simulink model "power_turbine_period2_1110_plots"  (R2025b)
settings: Solver=VariableStepAuto  StartTime=0.0  StopTime=100  RelTol=1e-3
undefined symbols (not defined in the file or in its folder): D1, Delta
libraries: spsThreePhaseBreakerLib x5, spsThreePhaseParallelRLCLoadLib x4, spsThreePhaseDynamicLoadLib x3, spsThreePhasePISectionLineLib x2, spsExcitationSystemLib x1, spsHydraulicTurbineandGovernorLib x1, spsLoadFlowBusLib x1, spsSynchronousMachinepuStandardLib x1, spsThreePhaseVIMeasurementLib x1, spsThreePhaseFaultLib x1, spsThreePhaseTransformerTwoWindingsLib x1, spsVoltageMeasurementLib x1
settings Model: Creator=Amaya  LastModifiedBy=Amaya

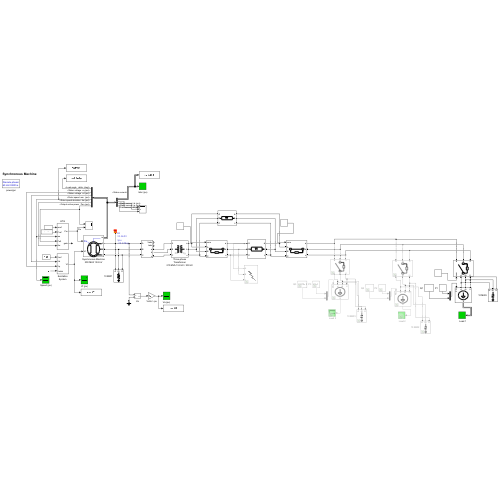
[thumbnail: Simulink's stored preview of the top-level diagram]
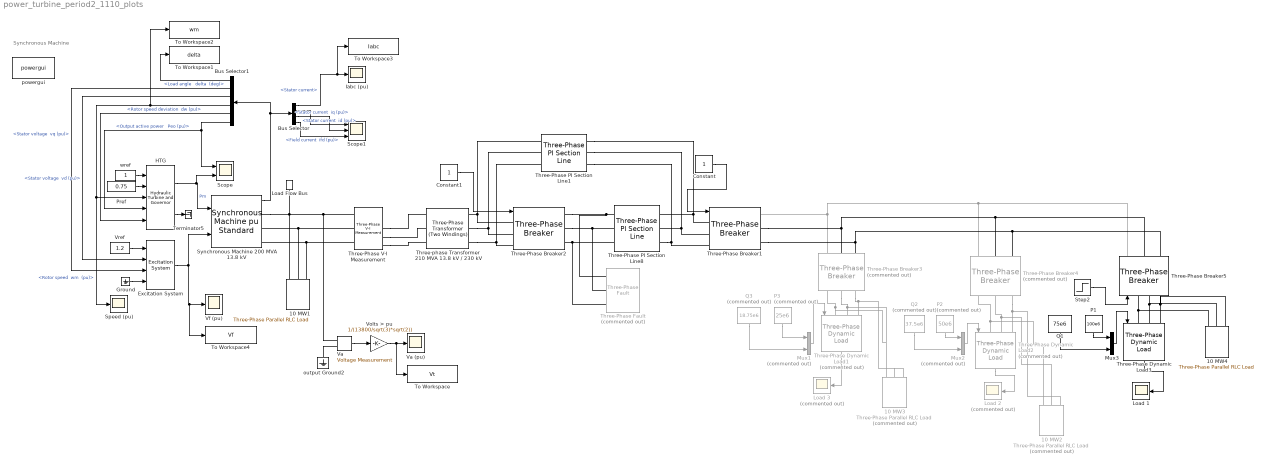
== system power_turbine_period2_1110_plots ==
  note: Synchronous Machine
  "  Load 1" : Scope
      settings: TimeSpan=2  ActiveDisplayYMinimum=-1.249999884558E+7  ActiveDisplayYMaximum=1.1249999987173E+8  DataLoggingVariableName=ScopeData3  DataLoggingSaveFormat=Array
  "  Load 2" : Scope  Commented=on
      settings: TimeSpan=2  ActiveDisplayYMinimum=-1.25E+7  ActiveDisplayYMaximum=1.125E+8  DataLoggingSaveFormat=Array
  "  Load 3" : Scope  Commented=on
      settings: TimeSpan=2  ActiveDisplayYMinimum=-1.25E+7  ActiveDisplayYMaximum=1.125E+8  DataLoggingVariableName=ScopeData2  DataLoggingSaveFormat=Array
  " Iabc (pu)" : Scope
      settings: TimeSpan=2  ActiveDisplayYMinimum=0.37186  ActiveDisplayYMaximum=0.41748  DataLoggingSaveFormat=Array
  " Speed (pu)" : Scope
      settings: TimeSpan=2  ActiveDisplayYMinimum=0.96201  ActiveDisplayYMaximum=1.29502  DataLoggingVariableName=ScopeData2  DataLoggingSaveFormat=Array
  10 MW1 : spsThreePhaseParallelRLCLoadLib/Three-Phase Parallel RLC Load  LConnTagsString=A|B|C  Configuration=Y (grounded)  NominalVoltage=230e3  Vabc=[1e3 1e3 1e3]  Vabcp=[1e3 1e3 1e3]  NominalFrequency=60  UnbalancedPower=off  ActivePower=5e6  InductivePower=0  CapacitivePower=0  Pabc=[10e3 9e3 11e3]  QLabc=[100 90 110]  QCabc=[100 90 110]  Pabcp=[10e3 9e3 11e3]  QLabcp=[100 90 110]  QCabcp=[100 90 110]  Measurements=None  LoadType=constant Z
  10 MW2 : spsThreePhaseParallelRLCLoadLib/Three-Phase Parallel RLC Load  Commented=on  LConnTagsString=A|B|C  Configuration=Y (grounded)  NominalVoltage=230e3  Vabc=[1e3 1e3 1e3]  Vabcp=[1e3 1e3 1e3]  NominalFrequency=60  UnbalancedPower=off  ActivePower=0  InductivePower=0  CapacitivePower=18.44e6  Pabc=[10e3 9e3 11e3]  QLabc=[100 90 110]  QCabc=[100 90 110]  Pabcp=[10e3 9e3 11e3]  QLabcp=[100 90 110]  QCabcp=[100 90 110]  Measurements=None  LoadType=constant Z
  10 MW3 : spsThreePhaseParallelRLCLoadLib/Three-Phase Parallel RLC Load  Commented=on  LConnTagsString=A|B|C  Configuration=Y (grounded)  NominalVoltage=230e3  Vabc=[1e3 1e3 1e3]  Vabcp=[1e3 1e3 1e3]  NominalFrequency=60  UnbalancedPower=off  ActivePower=0  InductivePower=0  CapacitivePower=9.21e6  Pabc=[10e3 9e3 11e3]  QLabc=[100 90 110]  QCabc=[100 90 110]  Pabcp=[10e3 9e3 11e3]  QLabcp=[100 90 110]  QCabcp=[100 90 110]  Measurements=None  LoadType=constant Z
  10 MW4 : spsThreePhaseParallelRLCLoadLib/Three-Phase Parallel RLC Load  LConnTagsString=A|B|C  Configuration=Y (grounded)  NominalVoltage=230e3  Vabc=[1e3 1e3 1e3]  Vabcp=[1e3 1e3 1e3]  NominalFrequency=60  UnbalancedPower=off  ActivePower=0  InductivePower=0  CapacitivePower=36.87e6  Pabc=[10e3 9e3 11e3]  QLabc=[100 90 110]  QCabc=[100 90 110]  Pabcp=[10e3 9e3 11e3]  QLabcp=[100 90 110]  QCabcp=[100 90 110]  Measurements=None  LoadType=constant Z
  Bus Selector : BusSelector  OutputSignals="Stator current,dq0 components.Stator current  id (pu),dq0 components.Stator current  iq (pu),dq0 components.Field current  ifd (pu)"
  Bus Selector1 : BusSelector  OutputSignals="Load angle   delta  (deg),dq0 components.Stator voltage  vq (pu),dq0 components.Stator voltage  vd (pu),Mechanical.Rotor speed  wm  (pu),Mechanical.Rotor speed deviation  dw (pu),Output active power   Peo (pu)"
  Constant : Constant
  Constant1 : Constant
  Excitation System : spsExcitationSystemLib/Excitation System  tr=20e-3  reg=[ 300, 0.001 ]  exc=[ 1, 0 ]  tgr=[ 0, 0 ]  damp=[ 0.001, 0.1 ]  sat=[ 0, 0 ]  lim=[ -1000, 1000, 0 ]  v0=[1,1.29071]
  Ground : Ground
  HTG : spsHydraulicTurbineandGovernorLib/Hydraulic Turbine and Governor  sm="[ 10/3  0.07 ]"  gate="[  0.01  0.97518  -0.1  0.1 ]"  reg="[  0.05  1.163  0.105  0  0.01  ]"  hyd="[  0  2.67  ]"  dref=0  po=0.751606
  Load Flow Bus : spsLoadFlowBusLib/Load Flow Bus  LConnTagsString=a  Phases=single  Connectors=on one side  ID=B1  Vbase=13.8e3  Vref=1  Vangle=0  VLF=1  VLFb=1  VLFc=1  angleLF=-23.67  angleLFb=0  angleLFc=0
      settings: AttributesFormatString=%<ID>\n%<Vbase>V\n%<VLF>pu\n%<angleLF>deg.
  Mux1 : Mux  Commented=on  Inputs=2
  Mux2 : Mux  Commented=on  Inputs=2
  Mux3 : Mux  Inputs=2
  P1 : Constant  Value=100e6
  P2 : Constant  Commented=on  Value=50e6
  P3 : Constant  Commented=on  Value=25e6
  Pref : Constant  Value=0.75
  Q1 : Constant  Value=75e6
  Q2 : Constant  Commented=on  Value=37.5e6
  Q3 : Constant  Commented=on  Value=18.75e6
  Scope : Scope  NumInputPorts=2
      settings: ActiveDisplayYMinimum=-11.7999  ActiveDisplayYMaximum=2.34274  DataLoggingVariableName=ScopeData4
  Scope1 : Scope  NumInputPorts=3
      settings: ActiveDisplayYMinimum=-1.06949  ActiveDisplayYMaximum=2.5715  DataLoggingVariableName=ScopeData4
  Step2 : Step  Time=0  SampleTime=0
  Synchronous Machine 200 MVA 13.8 kV : spsSynchronousMachinepuStandardLib/Synchronous Machine pu Standard  PresetModel=No  MechanicalLoad=Mechanical power Pm  ShowDetailedParameters=on  RotorType=Salient-pole  Units=per unit standard parameters  MeasurementBus=off  NominalParameters="[ 250E6  13800   60 ]"  Reactances1=[ 31 32 33 34 35 36 37 ]  Reactances2=[ 1.305, 0.296, 0.252, 0.474, 0.243, 0.18 ]  dAxisTimeConstants=Short-circuit  qAxisTimeConstants=Open-circuit  TimeConstants1=[]  TimeConstants2=[]  TimeConstants3=[]  TimeConstants4=[]  TimeConstants5=[ 1.01, 0.053, 0.1 ]  TimeConstants6=[]  TimeConstants7=[]  TimeConstants8=[]  StatorResistance=2.8544e-3  Mechanical=[ 3.2 0 2]  PolePairs=2  InitialConditions=[0 -94.2826 0.750185 0.750185 0.750185 -24.943 -144.943 95.057 1.29071]  SetSaturation=off  Saturation=[0.6404,0.7127,0.8441,0.9214,0.9956,1.082,1.19,1.316,1.457;0.7,0.7698,0.8872,0.9466,0.9969,1.046,1.1,1.151,1.201]  LoadFlowParameters=[1 150000000 0 0]  TsPowergui=0  TsBlock=-1  IterativeModel=Trapezoidal non iterative  IterativeDiscreteModel=Trapezoidal non iterative  BusType=PV  Pref=150000000  Qref=0  Qmin=-Inf  Qmax=Inf  PLF=0  QLF=0
  Terminator5 : Terminator
  Three-Phase Dynamic Load1 : spsThreePhaseDynamicLoadLib/Three-Phase Dynamic Load  Commented=on  NominalVoltage=[ 230e3 60 ]  ActiveReactivePowers=[25e6 18.75e6]  PositiveSequence=[0.994 -11.8]  ExternalControl=on  NpNq=[1.3 2]  TimeConstants="[0  0  0  0]"  MinimumVoltage=0.7  Tfilter=1e-4  LoadFlowParameters=[4,0,0,0,0]
      settings: LibrarySourceBlock=|
      | sps_lib/Passives/Three-Phase
      | Dynamic Load
  Three-Phase Dynamic Load2 : spsThreePhaseDynamicLoadLib/Three-Phase Dynamic Load  Commented=on  NominalVoltage=[ 230e3 60 ]  ActiveReactivePowers=[50e6 37.5e6]  PositiveSequence=[0.994 -11.8]  ExternalControl=on  NpNq=[1.3 2]  TimeConstants="[0  0  0  0]"  MinimumVoltage=0.7  Tfilter=1e-4  LoadFlowParameters=[4,0,0,0,0]
      settings: LibrarySourceBlock=|
      | sps_lib/Passives/Three-Phase
      | Dynamic Load
  Three-Phase Dynamic Load3 : spsThreePhaseDynamicLoadLib/Three-Phase Dynamic Load  NominalVoltage=[ 230e3 60 ]  ActiveReactivePowers=[100e6 75e6]  PositiveSequence=[0.994 -11.8]  ExternalControl=on  NpNq=[1.3 2]  TimeConstants="[0  0  0  0]"  MinimumVoltage=0.7  Tfilter=1e-4  LoadFlowParameters=[4,0,0,0,0]
      settings: LibrarySourceBlock=|
      | sps_lib/Passives/Three-Phase
      | Dynamic Load
  Three-Phase PI Section Line1 : spsThreePhasePISectionLineLib/Three-Phase PI Section Line  LConnTagsString=a|b|c  RConnTagsString=A|B|C  Length=125  Frequency=50  Resistances=[ 0.01273 0.3864]  Inductances="[ 0.9337e-3  4.1264e-3]"  Capacitances=[12.74e-9 7.751e-9]
  Three-Phase PI Section Line8 : spsThreePhasePISectionLineLib/Three-Phase PI Section Line  LConnTagsString=a|b|c  RConnTagsString=A|B|C  Length=125  Frequency=60  Resistances=[ 0.01273 0.3864]  Inductances="[ 0.9337e-3  4.1264e-3]"  Capacitances=[12.74e-9 7.751e-9]
  Three-Phase V-I Measurement : spsThreePhaseVIMeasurementLib/Three-Phase V-I Measurement  VoltageMeasurement=phase-to-ground  SetLabelV=off  LabelV=Vabc  Vpu=off  VpuLL=off  CurrentMeasurement=yes  SetLabelI=off  LabelI=Iabc  Ipu=off  Pbase=100e6  Vbase=500e3  OutputType=Complex  PhasorSimulation=on  PSBequivalent=0
  Three-Phase Breaker1 : spsThreePhaseBreakerLib/Three-Phase Breaker  InitialState=closed  SwitchA=on  SwitchB=on  SwitchC=on  SwitchTimes=[70.1 70+121/60]  External=on  BreakerResistance=0.01  SnubberResistance=1e6  SnubberCapacitance=inf  Measurements=None
  Three-Phase Breaker2 : spsThreePhaseBreakerLib/Three-Phase Breaker  InitialState=closed  SwitchA=on  SwitchB=on  SwitchC=on  SwitchTimes=[70.05 70.05+121/60]  External=on  BreakerResistance=0.01  SnubberResistance=1e6  SnubberCapacitance=inf  Measurements=None
  Three-Phase Breaker3 : spsThreePhaseBreakerLib/Three-Phase Breaker  Commented=on  InitialState=open  SwitchA=on  SwitchB=on  SwitchC=on  SwitchTimes=[100]  External=off  BreakerResistance=0.01  SnubberResistance=1e6  SnubberCapacitance=inf  Measurements=None
  Three-Phase Breaker4 : spsThreePhaseBreakerLib/Three-Phase Breaker  Commented=on  InitialState=open  SwitchA=on  SwitchB=on  SwitchC=on  SwitchTimes=[50]  External=off  BreakerResistance=0.01  SnubberResistance=1e6  SnubberCapacitance=inf  Measurements=None
  Three-Phase Breaker5 : spsThreePhaseBreakerLib/Three-Phase Breaker  InitialState=open  SwitchA=on  SwitchB=on  SwitchC=on  SwitchTimes="[7/60  121/60]"  External=on  BreakerResistance=0.01  SnubberResistance=1e6  SnubberCapacitance=inf  Measurements=None
  Three-Phase Fault : spsThreePhaseFaultLib/Three-Phase Fault  Commented=on  InitialStates=0  FaultA=on  FaultB=on  FaultC=on  GroundFault=on  SwitchTimes=[70 70.1]  External=off  SwitchStatus=NaN  FaultResistance=0.001  GroundResistance=1  SnubberResistance=1e6  SnubberCapacitance=inf  Measurements=None
  Three-phase Transformer 210 MVA 13.8 kV / 230 kV : spsThreePhaseTransformerTwoWindingsLib/Three-Phase Transformer (Two Windings)  Winding1Connection=Delta (D1)  Winding2Connection=Yg  CoreType=Three single-phase transformers  SetSaturation=off  Hysteresis=off  DataFile='hysteresis'  SetInitialFlux=off  Measurements=None  UNITS=pu  NominalPower=[ 210e6 60 ]  Winding1="[ 13.8e3 0.0027  0.08]"  Winding2=[ 230e3 0.0027 0.08]  Rm=500  Lm=500  L0=0.5  Saturation="[ 0,0  ;  0.005,1.2  ;  1.0,1.4 ]"  InitialFluxes=[ 0.8 , -0.8 , 0.7 ]  BreakLoop=off  DiscreteSolver=Trapezoidal iterative  DataType=off  TransfoNumber=0
  To Workspace : ToWorkspace  VariableName=Vt  SaveFormat=Structure With Time  SampleTime=-1
  To Workspace1 : ToWorkspace  VariableName=delta  SaveFormat=Structure With Time  SampleTime=-1
  To Workspace2 : ToWorkspace  VariableName=wm  SaveFormat=Structure With Time  SampleTime=-1
  To Workspace3 : ToWorkspace  VariableName=Iabc  SaveFormat=Structure With Time  SampleTime=-1
  To Workspace4 : ToWorkspace  VariableName=Vf  SaveFormat=Structure With Time  SampleTime=-1
  Va : spsVoltageMeasurementLib/Voltage Measurement  Tag=PoWeRsYsTeMmEaSuReMeNt  PhasorSimulation=on  OutputType=Magnitude  PSBequivalent=0
  Va (pu) : Scope
      settings: TimeSpan=2  ActiveDisplayYMinimum=0.99758  ActiveDisplayYMaximum=1.29648  DataLoggingVariableName=ScopeData3  DataLoggingSaveFormat=Array
  Vf (pu) : Scope
      settings: TimeSpan=2  ActiveDisplayYMinimum=-5.63103  ActiveDisplayYMaximum=28.67601  DataLoggingSaveFormat=Array
  Volts > pu : Gain  Gain=1/(13800/sqrt(3)*sqrt(2))  SaturateOnIntegerOverflow=on  OutDataTypeStr=Inherit: Same as input  ParamDataTypeStr=Inherit: Same as input
  Vref : Constant  Value=1.2
  output Ground2 : spsGroundLib/Ground  LConnTagsString=a
  powergui : spspowerguiLib/powergui  Priority=2  SimulationMode=Discrete phasor  SampleTime=50e-5  frequency=60  Iterations=50  frequencyindice=60  Pbase=100e6  ErrMax=0.0001  UnitsV=kV  UnitsW=MW  buscounter=0  FunctionMessages=off  echomessages=off  EnableUseOfTLC=off  CurrentSourceSwitches=off  DisableSnubberDevices=off  DisableRonSwitches=off  DisableVfSwitches=off  DisplayEquations=off  AutomaticDiscreteSolvers=off  SolverType=Tustin  Interpol=off  ExternalGateDelay=off  methode=off  Ts=0  x0status=blocks  SPID=on  SwTol=0  HookPort=off  NonlinearTolerance=1e-4  nMaxIteration=100  ContinueOnMaxIteration=off  RestoreLinks=warning  ResistiveCurrentMeasurement=off  Frange=logspace(0,3,50)  Ylog=off  Xlog=off  ShowGrid=off  save=off  variable=ZData  structure=0  ZoomFFT=on  StartTime=0.0  cycles=2  DisplayStyle=off  fundamental=60  FreqAxis=off  MaxFrequency=1000  frequencyindicesteady=1  RmsSteady=1  display=off
  wref : Constant
  wires:
  Excitation System/1 -> To Workspace4/1, Vf (pu)/1, Synchronous Machine 200 MVA 13.8 kV/2
  Bus Selector1/3 -> Excitation System/2  "<Stator voltage  vd (pu)>"
  Va/1 -> Volts > pu/1
  Bus Selector1/5 -> HTG/5  "<Rotor speed deviation  dw (pu)>"
  Ground/1 -> Excitation System/4
  Bus Selector1/6 -> Scope/1, HTG/4  "<Output active power   Peo (pu)>"
  Vref/1 -> Excitation System/1
  Synchronous Machine 200 MVA 13.8 kV/1 -> Bus Selector/1, Bus Selector1/1
  Bus Selector1/4 -> To Workspace2/1, HTG/3, " Speed (pu)"/1  "<Rotor speed  wm  (pu)>"
  Bus Selector1/2 -> Excitation System/3  "<Stator voltage  vq (pu)>"
  wref/1 -> HTG/1
  HTG/2 -> Terminator5/1
  Bus Selector/1 -> To Workspace3/1, " Iabc (pu)"/1  "<Stator current>"
  Volts > pu/1 -> To Workspace/1, Va (pu)/1
  Pref/1 -> HTG/2
  HTG/1 -> Scope/2, Synchronous Machine 200 MVA 13.8 kV/1  "Pm"
  Q3/1 -> Mux1/2
  Mux1/1 -> Three-Phase Dynamic Load1/1
  P3/1 -> Mux1/1
  Three-Phase Dynamic Load1/1 -> "  Load 3"/1
  Three-Phase Dynamic Load2/1 -> "  Load 2"/1
  P2/1 -> Mux2/1
  Mux2/1 -> Three-Phase Dynamic Load2/1
  Q2/1 -> Mux2/2
  Q1/1 -> Mux3/2
  Mux3/1 -> Three-Phase Dynamic Load3/1
  P1/1 -> Mux3/1
  Three-Phase Dynamic Load3/1 -> "  Load 1"/1
  Step2/1 -> Three-Phase Breaker5/1
  Constant/1 -> Three-Phase Breaker1/1
  Constant1/1 -> Three-Phase Breaker2/1
  Bus Selector/2 -> Scope1/1  "<Stator current  id (pu)>"
  Bus Selector/3 -> Scope1/2  "<Stator current  iq (pu)>"
  Bus Selector/4 -> Scope1/3  "<Field current  ifd (pu)>"
  Bus Selector1/1 -> To Workspace1/1  "<Load angle   delta  (deg)>"
  connections:
  Load Flow Bus/LConn1 -- 10 MW1/LConn1 -- Synchronous Machine 200 MVA 13.8 kV/RConn1 -- Three-Phase V-I Measurement/LConn1 -- Va/LConn1
  10 MW1/LConn3 -- Synchronous Machine 200 MVA 13.8 kV/RConn3 -- Three-Phase V-I Measurement/LConn3
  10 MW1/LConn2 -- Three-Phase V-I Measurement/LConn2 -- Synchronous Machine 200 MVA 13.8 kV/RConn2
  output Ground2/LConn1 -- Va/LConn2
  Three-Phase Breaker1/LConn2 -- Three-Phase PI Section Line1/RConn2 -- Three-Phase PI Section Line8/RConn2
  Three-Phase Breaker1/LConn1 -- Three-Phase PI Section Line1/RConn1 -- Three-Phase PI Section Line8/RConn1
  Three-Phase PI Section Line8/RConn3 -- Three-Phase PI Section Line1/RConn3 -- Three-Phase Breaker1/LConn3
  Three-Phase Breaker2/RConn1 -- Three-Phase Fault/LConn1 -- Three-Phase PI Section Line8/LConn1
  Three-Phase Breaker2/RConn2 -- Three-Phase PI Section Line8/LConn2 -- Three-Phase Fault/LConn2
  Three-Phase Breaker2/RConn3 -- Three-Phase PI Section Line8/LConn3 -- Three-Phase Fault/LConn3
  Three-phase Transformer 210 MVA 13.8 kV / 230 kV/RConn1 -- Three-Phase PI Section Line1/LConn1 -- Three-Phase Breaker2/LConn1
  Three-phase Transformer 210 MVA 13.8 kV / 230 kV/RConn2 -- Three-Phase PI Section Line1/LConn2 -- Three-Phase Breaker2/LConn2
  Three-phase Transformer 210 MVA 13.8 kV / 230 kV/RConn3 -- Three-Phase PI Section Line1/LConn3 -- Three-Phase Breaker2/LConn3
  Three-Phase Breaker4/RConn1 -- Three-Phase Breaker5/RConn1 -- Three-Phase Breaker3/RConn1 -- Three-Phase Breaker1/RConn1
  Three-Phase Breaker1/RConn2 -- Three-Phase Breaker5/RConn2 -- Three-Phase Breaker4/RConn2 -- Three-Phase Breaker3/RConn2
  Three-Phase Breaker1/RConn3 -- Three-Phase Breaker5/RConn3 -- Three-Phase Breaker4/RConn3 -- Three-Phase Breaker3/RConn3
  Three-Phase Dynamic Load1/LConn1 -- 10 MW3/LConn1 -- Three-Phase Breaker3/LConn1
  Three-Phase Breaker3/LConn2 -- 10 MW3/LConn2 -- Three-Phase Dynamic Load1/LConn2
  Three-Phase Breaker3/LConn3 -- 10 MW3/LConn3 -- Three-Phase Dynamic Load1/LConn3
  Three-Phase Dynamic Load2/LConn1 -- 10 MW2/LConn1 -- Three-Phase Breaker4/LConn1
  Three-Phase Dynamic Load2/LConn2 -- 10 MW2/LConn2 -- Three-Phase Breaker4/LConn2
  Three-Phase Dynamic Load3/LConn2 -- 10 MW4/LConn2 -- Three-Phase Breaker5/LConn2
  Three-Phase Dynamic Load3/LConn1 -- 10 MW4/LConn1 -- Three-Phase Breaker5/LConn1
  Three-Phase Dynamic Load3/LConn3 -- 10 MW4/LConn3 -- Three-Phase Breaker5/LConn3
  Three-Phase V-I Measurement/RConn1 -- Three-phase Transformer 210 MVA 13.8 kV / 230 kV/LConn1
  Three-Phase V-I Measurement/RConn2 -- Three-phase Transformer 210 MVA 13.8 kV / 230 kV/LConn2
  Three-Phase V-I Measurement/RConn3 -- Three-phase Transformer 210 MVA 13.8 kV / 230 kV/LConn3
  Three-Phase Breaker4/LConn3 -- 10 MW2/LConn3 -- Three-Phase Dynamic Load2/LConn3
